simulink model "PID2Nonlinear"  (R2020b)
settings: Solver=VariableStepAuto  StartTime=0.0  StopTime=10  RelTol=1e-3
libraries: pid_lib x7, simulink x7
settings Model: Creator=arthur  LastModifiedBy=arthur

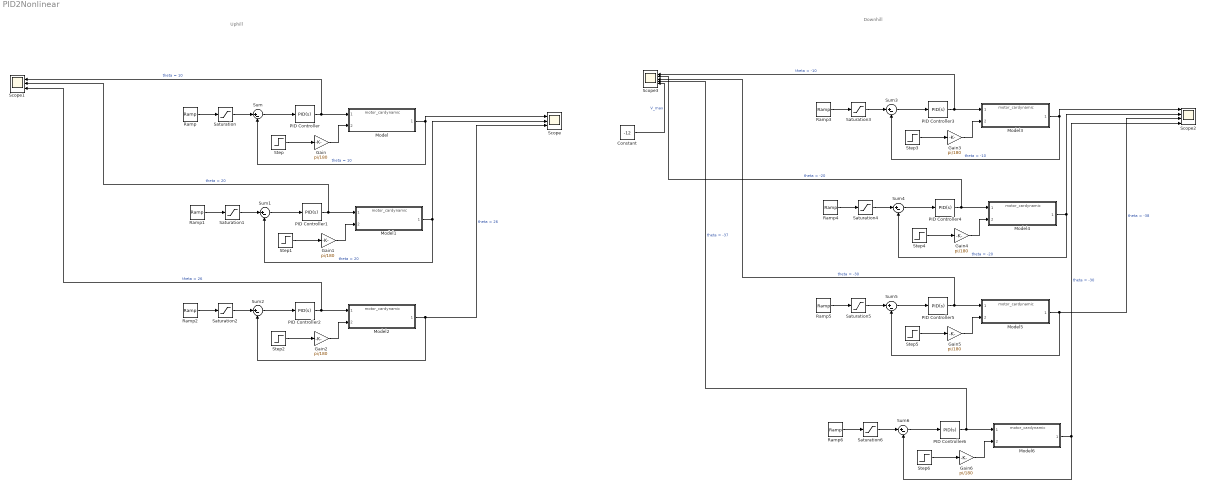
== system PID2Nonlinear ==
  note: Uphill
  note: Downhill
  Constant : Constant  Value=-12
  Gain{,1..6} (7 alike) : Gain  Gain=pi/180
  Model{,1..6} (7 alike) : ModelReference  ModelNameDialog=motor_cardynamic.slx  SimulationMode=Normal  ModelReferenceVersion=1.10
  PID Controller{,1..6} (7 alike) : pid_lib/PID Controller  Controller=PID  Form=Parallel  TimeDomain=Continuous-time  UseExternalTs=off  SampleTime=-1  IntegratorMethod=Forward Euler  FilterMethod=Forward Euler  ControllerParametersSource=internal  P=11  I=13.2  D=2.2  UseFilter=on  N=100  TunerSelectOption=Transfer Function Based (PID Tuner App)  InitialConditionSource=internal  InitialConditionForIntegrator=0  InitialConditionForFilter=0  DifferentiatorICPrevScaledInput=0  ExternalReset=none  TrackingMode=off  Kt=1  LimitOutput=off  SatLimitsSource=internal  UpperSaturationLimit=inf  LowerSaturationLimit=-inf  LinearizeAsGain=on  AntiWindupMode=none  Kb=1  POutMin=[]  POutMax=[]  IOutMin=[]  IOutMax=[]  DOutMin=[]  DOutMax=[]  NOutMin=[]  NOutMax=[]  SumOutMin=[]  SumOutMax=[]  SaturationOutMin=[]  SaturationOutMax=[]  PParamMin=[]  PParamMax=[]  IParamMin=[]  IParamMax=[]  DParamMin=[]  DParamMax=[]  NParamMin=[]  NParamMax=[]  KbParamMin=[]  KbParamMax=[]  KtParamMin=[]  KtParamMax=[]  KbOutMin=[]  KbOutMax=[]  KtOutMin=[]  KtOutMax=[]  IntegratorOutMin=[]  IntegratorOutMax=[]  FilterOutMin=[]  FilterOutMax=[]  SumI1OutMin=[]  SumI1OutMax=[]  SumI2OutMin=[]  SumI2OutMax=[]  SumI3OutMin=[]  SumI3OutMax=[]  SumI4OutMin=[]  SumI4OutMax=[]  SumDOutMin=[]  SumDOutMax=[]  DifferentiatorOutMin=[]  DifferentiatorOutMax=[]  FilterDiffOutCoefMin=[]  FilterDiffOutCoefMax=[]  ReciprocalOutMin=[]  ReciprocalOutMax=[]  SumDenOutMin=[]  SumDenOutMax=[]  SumNumOutMin=[]  SumNumOutMax=[]  DivideOutMin=[]  DivideOutMax=[]  UdiffTsProdOutMin=[]  UdiffTsProdOutMax=[]  NTsProdOutMin=[]  NTsProdOutMax=[]  UintegralTsProdOutMin=[]  UintegralTsProdOutMax=[]  UngainTsProdOutMin=[]  UngainTsProdOutMax=[]  IntegratorContinuousStateAttributes=''  IntegratorStateMustResolveToSignalObject=off  IntegratorRTWStateStorageClass=Auto  FilterContinuousStateAttributes=''  FilterStateMustResolveToSignalObject=off  FilterRTWStateStorageClass=Auto  ParallelPVariant=InternalParameters  IdealPVariant=Disabled  IVariant=InternalParameters  DVariant=InternalParameters  IntegratorVariant=Continuous  SatVariant=Disabled  AWVariant=Passthrough  PCopyVariant=Disabled  TRVariant=Disabled  FdbkBlocksVariant=Forward  IdealPFdbkVariant=Disabled  SatFdbkVariant=Disabled  DerivativeFilterVariant=ContFilter  NVariant=InternalParameters  NCopyVariant=Disabled  FilterICVariant=InternalICsFilter  IntegratorICVariant=InternalICs  ExternalResetVariant=Disabled  TRSumVariant=Passthrough  SumFdbkVariant=Disabled  SumVariant=Sum_PID  TsampFilterVariant=InternalTs  TsampNgainVariant=Passthrough  TsampIntegralVariant=Passthrough  ExternalSaturationOutDataTypeStr=Inherit: Same as second input
  Ramp{,1..6} (7 alike) : simulink/Sources/Ramp  slope=5  start=0  InitialOutput=0
  Saturation{,1..6} (7 alike) : Saturate  UpperLimit=1  LowerLimit=0
  Scope : Scope  NumInputPorts=3
  Scope1 : Scope  NumInputPorts=3
  Scope2 : Scope  NumInputPorts=4
  Scope3 : Scope  NumInputPorts=5
  Step : Step  Time=5  After=10  SampleTime=0
  Step1 : Step  Time=5  After=20  SampleTime=0
  Step2 : Step  Time=5  After=26  SampleTime=0
  Step3 : Step  Time=5  After=-10  SampleTime=0
  Step4 : Step  Time=5  After=-20  SampleTime=0
  Step5 : Step  Time=5  After=-30  SampleTime=0
  Step6 : Step  Time=5  After=-37  SampleTime=0
  Sum{,1..6} (7 alike) : Sum  Inputs=|+-
  wires:
  Gain/1 -> Model/2
  Model/1 -> Sum/2, Scope/1  "theta = 10"
  Saturation/1 -> Sum/1
  Ramp/1 -> Saturation/1
  Sum/1 -> PID Controller/1
  PID Controller/1 -> Scope1/1, Model/1  "theta = 10"
  Step/1 -> Gain/1
  Model1/1 -> Scope/2, Sum1/2  "theta = 20"
  Ramp1/1 -> Saturation1/1
  PID Controller1/1 -> Scope1/2, Model1/1  "theta = 20"
  Saturation1/1 -> Sum1/1
  Gain1/1 -> Model1/2
  Sum1/1 -> PID Controller1/1
  Step1/1 -> Gain1/1
  Model2/1 -> Scope/3, Sum2/2  "theta = 26"
  Ramp2/1 -> Saturation2/1
  PID Controller2/1 -> Scope1/3, Model2/1  "theta = 26"
  Saturation2/1 -> Sum2/1
  Gain2/1 -> Model2/2
  Sum2/1 -> PID Controller2/1
  Step2/1 -> Gain2/1
  Model3/1 -> Sum3/2, Scope2/1  "theta = -10"
  Saturation3/1 -> Sum3/1
  Saturation5/1 -> Sum5/1
  Ramp4/1 -> Saturation4/1
  Gain3/1 -> Model3/2
  PID Controller3/1 -> Scope3/1, Model3/1  "theta = -10"
  PID Controller4/1 -> Scope3/2, Model4/1  "theta = -20"
  Ramp3/1 -> Saturation3/1
  Sum3/1 -> PID Controller3/1
  Sum4/1 -> PID Controller4/1
  Step3/1 -> Gain3/1
  Ramp5/1 -> Saturation5/1
  Model4/1 -> Scope2/2, Sum4/2  "theta = -20"
  Gain4/1 -> Model4/2
  Saturation4/1 -> Sum4/1
  Step4/1 -> Gain4/1
  Step5/1 -> Gain5/1
  Model5/1 -> Scope2/3, Sum5/2  "theta = -38"
  Sum5/1 -> PID Controller5/1
  Gain5/1 -> Model5/2
  PID Controller5/1 -> Scope3/3, Model5/1  "theta = -30"
  Gain6/1 -> Model6/2
  PID Controller6/1 -> Scope3/4, Model6/1  "theta = -37"
  Saturation6/1 -> Sum6/1
  Model6/1 -> Scope2/4, Sum6/2  "theta = -30"
  Step6/1 -> Gain6/1
  Ramp6/1 -> Saturation6/1
  Sum6/1 -> PID Controller6/1
  Constant/1 -> Scope3/5  "V_max"
